simulink model "pato4CM00_23hz"  (R2015b)
settings: Solver=FixedStepDiscrete  StartTime=0.0  StopTime=1000  FixedStep=1/2048  RelTol=1e-3
settings Model: SimulationMode=external  ExtModeAutoUpdateStatusClock=off  Creator=root  LastModifiedBy=root
settings DataIOCC: LimitDataPoints=off  SaveFormat=Array  SignalLoggingSaveFormat=ModelDataLogs
settings OptimizationCC: ExpressionDepthLimit=2147483647  InitFltsAndDblsToZero=on
settings DebuggingCC: UnderspecifiedInitializationDetection=Classic  MergeDetectMultiDrivingBlocksExec=none  SolverPrmCheckMsg=warning  FcnCallInpInsideContextMsg=UseLocalSettings  StateNameClashWarn=warning
settings HardwareCC: ProdBitPerPointer=32  ProdLargestAtomicFloat=None  ProdIntDivRoundTo=Undefined  ProdEndianess=Unspecified  ProdWordSize=32  ProdHWDeviceType=32-bit Generic
settings RTWCC: SystemTargetFile=ectarget.tlc  MakeCommand="make_rtw OPTS=\"-DNETIF_ID=2\""  TemplateMakefile=ec_unix.tmf  Description=EtherCAT Real-Time Target for SOEM (IME Technologies 2008)
settings GRTTargetCC: GeneratePreprocessorConditionals=Disable all  CombineOutputUpdateFcns=off  GRTInterface=on  UseToolchainInfoCompliant=off  ExtMode=on
settings ConfigComp: CovModelRefEnable=Off  CovSFcnEnable=off

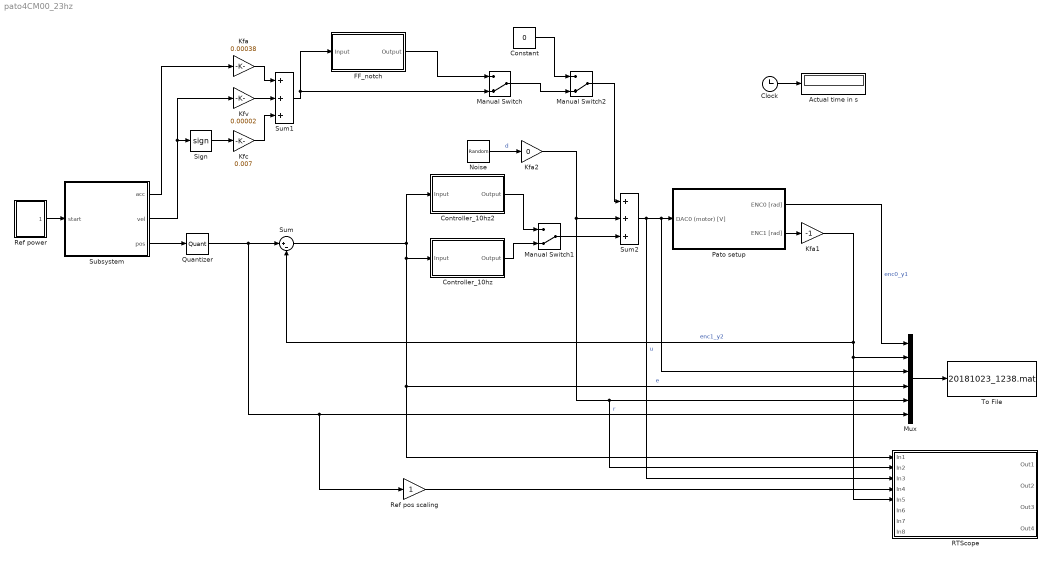
== system pato4CM00_23hz ==
  Actual time in s : Display
  Clock : Clock
  Constant : Constant  Value=0
  Controller_10hz : Subsystem  mask(Controller){Kp=100, Kv=0.005, notch_zeros=59, notch_damping_zeros=0.03, notch_poles=59, notch_damping_poles=0.5, roll_off_poles=200, roll_off_damping_poles=0.5}
      mask prompts: notch_zeros "Notch zeros [Hz]"; notch_damping_zeros "Notch damping zeros [-]"; notch_poles "Notch poles [Hz]"; notch_damping_poles "Notch damping poles [-]"; roll_off_poles "Roll-off poles [Hz]"; roll_off_damping_poles "Roll-off damping poles [-]"
      mask help:
      | The controller consists of three filters: a Kp/Kv, a notch and a roll-off filter.
      | You can edit the parameters below.
  Controller_10hz2 : Subsystem  mask(Controller){Kp=100, Kv=0.005, notch_zeros=59, notch_damping_zeros=0.03, notch_poles=59, notch_damping_poles=0.5, roll_off_poles=200, roll_off_damping_poles=0.5}
      mask prompts: notch_zeros "Notch zeros [Hz]"; notch_damping_zeros "Notch damping zeros [-]"; notch_poles "Notch poles [Hz]"; notch_damping_poles "Notch damping poles [-]"; roll_off_poles "Roll-off poles [Hz]"; roll_off_damping_poles "Roll-off damping poles [-]"
      mask help:
      | The controller consists of three filters: a Kp/Kv, a notch and a roll-off filter.
      | You can edit the parameters below.
  FF_notch : Subsystem  mask(Controller){Kp=100, Kv=0.005, notch_zeros=59, notch_damping_zeros=0.03, notch_poles=59, notch_damping_poles=0.5, roll_off_poles=200, roll_off_damping_poles=0.5}
      mask prompts: notch_zeros "Notch zeros [Hz]"; notch_damping_zeros "Notch damping zeros [-]"; notch_poles "Notch poles [Hz]"; notch_damping_poles "Notch damping poles [-]"; roll_off_poles "Roll-off poles [Hz]"; roll_off_damping_poles "Roll-off damping poles [-]"
      mask help:
      | The controller consists of three filters: a Kp/Kv, a notch and a roll-off filter.
      | You can edit the parameters below.
  Kfa : Gain  Gain=0.00038  SaturateOnIntegerOverflow=on  OutDataTypeStr=Inherit: Same as input  ParamDataTypeStr=Inherit: Same as input
  Kfa1 : Gain  Gain=-1  SaturateOnIntegerOverflow=on  OutDataTypeStr=Inherit: Same as input  ParamDataTypeStr=Inherit: Same as input
  Kfa2 : Gain  Gain=0  SaturateOnIntegerOverflow=on  OutDataTypeStr=Inherit: Same as input  ParamDataTypeStr=Inherit: Same as input
  Kfc : Gain  Gain=0.007  SaturateOnIntegerOverflow=on  OutDataTypeStr=Inherit: Same as input  ParamDataTypeStr=Inherit: Same as input
  Kfv : Gain  Gain=0.00002  SaturateOnIntegerOverflow=on  OutDataTypeStr=Inherit: Same as input  ParamDataTypeStr=Inherit: Same as input
  Manual Switch : ManualSwitch  CurrentSetting=0
  Manual Switch1 : ManualSwitch  CurrentSetting=0
  Manual Switch2 : ManualSwitch  CurrentSetting=0
  Mux : Mux  Inputs=6
  Noise : RandomNumber  Variance=0.1  SampleTime=0
  Pato setup : Subsystem  mask(Encoders){}
      mask help: Inc encoder positions 1-2 [rad] (see connector pannel).
  Quantizer : Quantizer  QuantizationInterval=(2*pi)/(500*4)
  RTScope : Subsystem  mask(RTScope){}
      settings: OpenFcn=rtscope
      mask Display: image(imread('rtscope2.jpg'))
  Ref pos scaling : Gain  SaturateOnIntegerOverflow=on  OutDataTypeStr=Inherit: Same as input  ParamDataTypeStr=Inherit: Same as input
  Ref power : Subsystem  mask(On/Off Switch){stat=On}
      mask prompts: stat "Switch"
      mask TypeOptions stat: On | Off
  Sign : Signum
  Subsystem : Subsystem  mask(Ref3){}
      settings: OpenFcn=global ref_part; cb_axes 1
      mask Display: disp('Ref3');
  Sum : Sum  Inputs=|+-  SaturateOnIntegerOverflow=on  InputSameDT=on  OutDataTypeStr=Inherit: Same as first input
  Sum1 : Sum  Description=sumff  Inputs=+++  SaturateOnIntegerOverflow=on  InputSameDT=on  OutDataTypeStr=Inherit: Same as first input
  Sum2 : Sum  Description=sumff  Inputs=+++  SaturateOnIntegerOverflow=on  InputSameDT=on  OutDataTypeStr=Inherit: Same as first input
  To File : ToFile  Filename=20181023_1238.mat
  wires:
  Subsystem/1(acc) -> Kfa/1
  Sum/1 -> Controller_10hz2/1(Input), Mux/4, RTScope/1(In1), Controller_10hz/1(Input)  "e"
  Sign/1 -> Kfc/1
  Ref power/1(On/Off) -> Subsystem/1(start)
  Ref pos scaling/1 -> RTScope/4(In4)
  Sum2/1 -> RTScope/3(In3), Mux/3, Pato setup/1(DAC0 (motor) [V])  "u"
  Subsystem/3(pos) -> Quantizer/1
  Subsystem/2(vel) -> Kfv/1, Sign/1
  Clock/1 -> Actual time in s/1
  Quantizer/1 -> Sum/1, Mux/6, Ref pos scaling/1  "r"
  Pato setup/2(ENC1 [rad]) -> Kfa1/1
  Kfa1/1 -> Sum/2, RTScope/5(In5), Mux/2  "enc1_y2"
  Mux/1 -> To File/1
  Pato setup/1(ENC0 [rad]) -> Mux/1  "enc0_y1"
  Kfa2/1 -> RTScope/2(In2), Mux/5, Sum2/2
  Noise/1 -> Kfa2/1  "d"
  Kfc/1 -> Sum1/3
  Kfv/1 -> Sum1/2
  Kfa/1 -> Sum1/1
  Sum1/1 -> FF_notch/1(Input), Manual Switch/2
  Manual Switch1/1 -> Sum2/3
  Manual Switch/1 -> Manual Switch2/2
  Manual Switch2/1 -> Sum2/1
  Constant/1 -> Manual Switch2/1
  Controller_10hz/1(Output) -> Manual Switch1/2
  Controller_10hz2/1(Output) -> Manual Switch1/1
  FF_notch/1(Output) -> Manual Switch/1

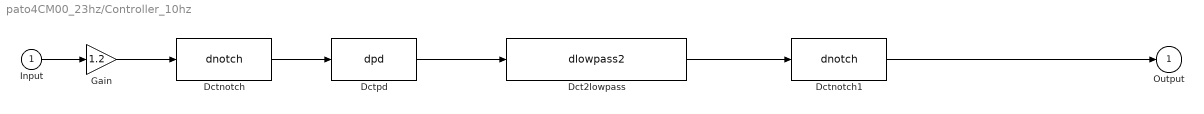
== system pato4CM00_23hz/Controller_10hz ==
  Input : Inport
  Dct2lowpass : S-Function  FunctionName=dlowpass2  Parameters=[f_den b_den 0.001]  SFunctionDeploymentMode=off  EnableBusSupport=off  mask(dctools){f_den=100, b_den=0.7}
      mask prompts: f_den "Pole [Hz]"; b_den "Damping pole [-]"
      mask help: This block implements a discrete time 2nd order lowpass filter.
      mask Display: disp('DCT 2nd order lowpass')
  Dctnotch : S-Function  FunctionName=dnotch  Parameters=[f_num b_num f_den b_den 0.001]  SFunctionDeploymentMode=off  EnableBusSupport=off  mask(dctools){f_num=58, b_num=0.005, f_den=59, b_den=0.5}
      mask prompts: f_num "Zero [Hz]"; b_num "Damping zero [-]"; f_den "Pole [Hz]"; b_den "Damping pole [-]"
      mask help: This block implements a dicrete time 2nd order notch filter.
      mask Display: disp('DCT notch')
  Dctnotch1 : S-Function  FunctionName=dnotch  Parameters=[f_num b_num f_den b_den 0.001]  SFunctionDeploymentMode=off  EnableBusSupport=off  mask(dctools){f_num=5, b_num=1, f_den=5, b_den=1}
      mask prompts: f_num "Zero [Hz]"; b_num "Damping zero [-]"; f_den "Pole [Hz]"; b_den "Damping pole [-]"
      mask help: This block implements a dicrete time 2nd order notch filter.
      mask Display: disp('DCT notch')
  Dctpd : S-Function  FunctionName=dpd  Parameters=[kp kv 0.001]  SFunctionDeploymentMode=off  EnableBusSupport=off  mask(dctools){kp=1, kv=0.03}
      mask help: This block implements a discrete time pd filter.
      mask Display: disp('DCT pd')
  Gain : Gain  Gain=1.2
  Output : Outport
  wires:
  Input/1 -> Gain/1
  Dct2lowpass/1 -> Dctnotch1/1
  Gain/1 -> Dctnotch/1
  Dctnotch/1 -> Dctpd/1
  Dctpd/1 -> Dct2lowpass/1
  Dctnotch1/1 -> Output/1

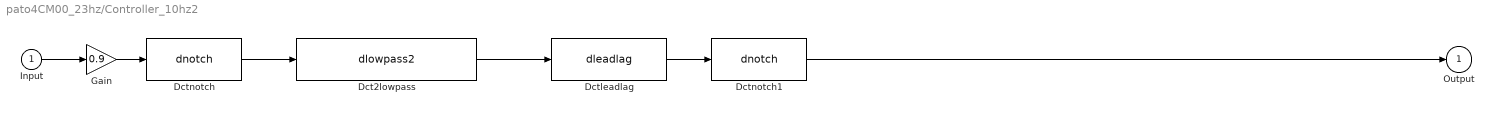
== system pato4CM00_23hz/Controller_10hz2 ==
  Input : Inport
  Dct2lowpass : S-Function  FunctionName=dlowpass2  Parameters=[f_den b_den 0.001]  SFunctionDeploymentMode=off  EnableBusSupport=off  mask(dctools){f_den=100, b_den=0.7}
      mask prompts: f_den "Pole [Hz]"; b_den "Damping pole [-]"
      mask help: This block implements a discrete time 2nd order lowpass filter.
      mask Display: disp('DCT 2nd order lowpass')
  Dctleadlag : S-Function  FunctionName=dleadlag  Parameters=[f_num f_den 0.001]  SFunctionDeploymentMode=off  EnableBusSupport=off  mask(dctools){f_num=11, f_den=30}
      mask prompts: f_num "Zero [Hz]"; f_den "Pole [Hz]"
      mask help: This block implements a discrete time leadlag filter.
      mask Display: disp('DCT leadlag')
  Dctnotch : S-Function  FunctionName=dnotch  Parameters=[f_num b_num f_den b_den 0.001]  SFunctionDeploymentMode=off  EnableBusSupport=off  mask(dctools){f_num=25.3, b_num=0.07, f_den=60, b_den=0.35}
      mask prompts: f_num "Zero [Hz]"; b_num "Damping zero [-]"; f_den "Pole [Hz]"; b_den "Damping pole [-]"
      mask help: This block implements a dicrete time 2nd order notch filter.
      mask Display: disp('DCT notch')
  Dctnotch1 : S-Function  FunctionName=dnotch  Parameters=[f_num b_num f_den b_den 0.001]  SFunctionDeploymentMode=off  EnableBusSupport=off  mask(dctools){f_num=5.5, b_num=0.6, f_den=7, b_den=1}
      mask prompts: f_num "Zero [Hz]"; b_num "Damping zero [-]"; f_den "Pole [Hz]"; b_den "Damping pole [-]"
      mask help: This block implements a dicrete time 2nd order notch filter.
      mask Display: disp('DCT notch')
  Gain : Gain  Gain=0.9
  Output : Outport
  wires:
  Input/1 -> Gain/1
  Gain/1 -> Dctnotch/1
  Dctnotch/1 -> Dct2lowpass/1
  Dctnotch1/1 -> Output/1
  Dct2lowpass/1 -> Dctleadlag/1
  Dctleadlag/1 -> Dctnotch1/1

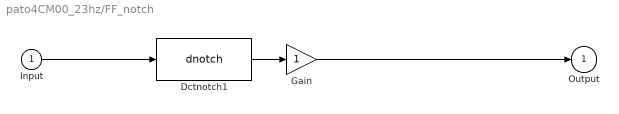
== system pato4CM00_23hz/FF_notch ==
  Input : Inport
  Dctnotch1 : S-Function  FunctionName=dnotch  Parameters=[f_num b_num f_den b_den 0.001]  SFunctionDeploymentMode=off  EnableBusSupport=off  mask(dctools){f_num=58, b_num=0.1, f_den=58, b_den=0.5}
      mask prompts: f_num "Zero [Hz]"; b_num "Damping zero [-]"; f_den "Pole [Hz]"; b_den "Damping pole [-]"
      mask help: This block implements a dicrete time 2nd order notch filter.
      mask Display: disp('DCT notch')
  Gain : Gain
  Output : Outport
  wires:
  Input/1 -> Dctnotch1/1
  Dctnotch1/1 -> Gain/1
  Gain/1 -> Output/1

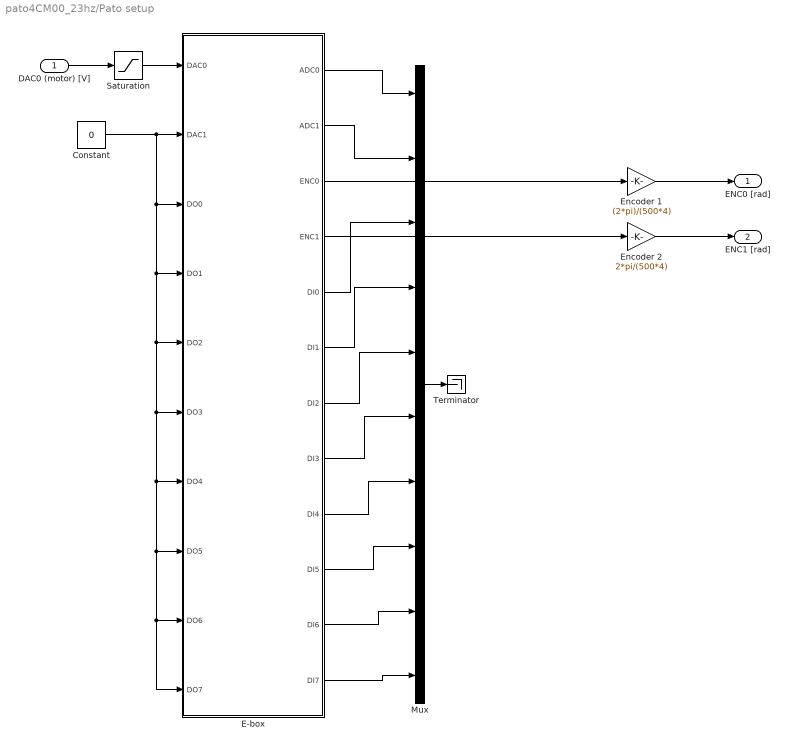
== system pato4CM00_23hz/Pato setup ==
  DAC0 (motor) [V] : Inport
  Constant : Constant  Value=0
  E-box : Subsystem  mask(E-box){link_id=0}
      mask prompts: link_id "Link id (>=0)"
  Encoder 1 : Gain  Gain=(2*pi)/(500*4)  SaturateOnIntegerOverflow=on  OutDataTypeStr=Inherit: Same as input  ParamDataTypeStr=Inherit: Same as input
  Encoder 2 : Gain  Gain=2*pi/(500*4)  SaturateOnIntegerOverflow=on  OutDataTypeStr=Inherit: Same as input  ParamDataTypeStr=Inherit: Same as input
  Mux : Mux  Inputs=10
  Saturation : Saturate  UpperLimit=2.5  LowerLimit=-2.5
  Terminator : Terminator
  ENC0 [rad] : Outport
  ENC1 [rad] : Outport  Port=2
  wires:
  E-box/3(ENC0) -> Encoder 1/1
  Encoder 1/1 -> ENC0 [rad]/1
  Encoder 2/1 -> ENC1 [rad]/1
  DAC0 (motor) [V]/1 -> Saturation/1
  Constant/1 -> E-box/2(DAC1), E-box/3(DO0), E-box/4(DO1), E-box/5(DO2), E-box/6(DO3), E-box/7(DO4), E-box/8(DO5), E-box/9(DO6), E-box/10(DO7)
  E-box/4(ENC1) -> Encoder 2/1
  E-box/1(ADC0) -> Mux/1
  E-box/2(ADC1) -> Mux/2
  E-box/5(DI0) -> Mux/3
  E-box/6(DI1) -> Mux/4
  E-box/7(DI2) -> Mux/5
  E-box/8(DI3) -> Mux/6
  E-box/9(DI4) -> Mux/7
  E-box/10(DI5) -> Mux/8
  E-box/11(DI6) -> Mux/9
  E-box/12(DI7) -> Mux/10
  Mux/1 -> Terminator/1
  Saturation/1 -> E-box/1(DAC0)

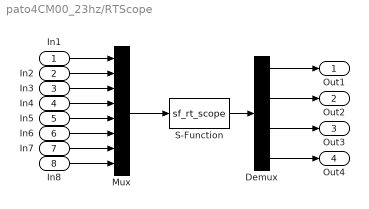
== system pato4CM00_23hz/RTScope ==
  In1 : Inport
  In2 : Inport  Port=2
  In3 : Inport  Port=3
  In4 : Inport  Port=4
  In5 : Inport  Port=5
  In6 : Inport  Port=6
  In7 : Inport  Port=7
  In8 : Inport  Port=8
  Demux : Demux
  Mux : Mux  Inputs=8
  S-Function : S-Function  FunctionName=sf_rt_scope  Parameters=4096  SFunctionDeploymentMode=off  EnableBusSupport=off
  Out1 : Outport
  Out2 : Outport  Port=2
  Out3 : Outport  Port=3
  Out4 : Outport  Port=4
  wires:
  In8/1 -> Mux/8
  In7/1 -> Mux/7
  In6/1 -> Mux/6
  In5/1 -> Mux/5
  In4/1 -> Mux/4
  In3/1 -> Mux/3
  In2/1 -> Mux/2
  In1/1 -> Mux/1
  Demux/4 -> Out4/1
  Demux/3 -> Out3/1
  Demux/2 -> Out2/1
  Demux/1 -> Out1/1
  S-Function/1 -> Demux/1
  Mux/1 -> S-Function/1

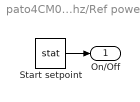
== system pato4CM00_23hz/Ref power ==
  Start setpoint : Constant  Value=stat
  On/Off : Outport
  wires:
  Start setpoint/1 -> On/Off/1

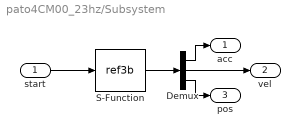
== system pato4CM00_23hz/Subsystem ==
  start : Inport
  Demux : Demux  Outputs=3
  S-Function : S-Function  FunctionName=ref3b  Parameters=ref_part  SFunctionDeploymentMode=off  EnableBusSupport=off
      settings: OpenFcn=global ref_part; r3g_main
  acc : Outport
  vel : Outport  Port=2
  pos : Outport  Port=3
  wires:
  S-Function/1 -> Demux/1
  Demux/1 -> acc/1
  Demux/2 -> vel/1
  Demux/3 -> pos/1
  start/1 -> S-Function/1

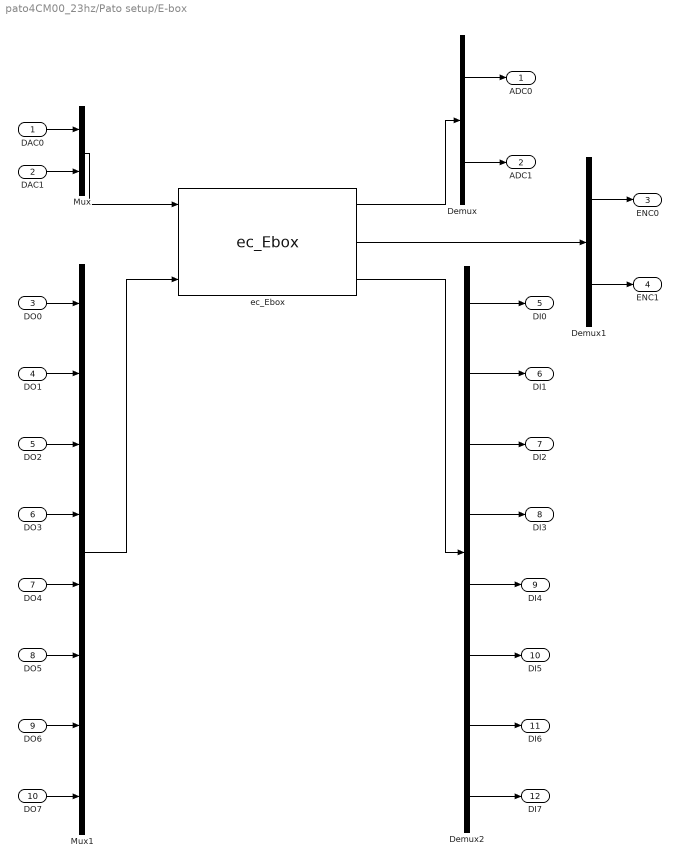
== system pato4CM00_23hz/Pato setup/E-box ==
  DAC0 : Inport
  DAC1 : Inport  Port=2
  DO0 : Inport  Port=3
  DO1 : Inport  Port=4
  DO2 : Inport  Port=5
  DO3 : Inport  Port=6
  DO4 : Inport  Port=7
  DO5 : Inport  Port=8
  DO6 : Inport  Port=9
  DO7 : Inport  Port=10
  Demux : Demux  Outputs=2
  Demux1 : Demux  Outputs=2
  Demux2 : Demux  Outputs=8
  Mux : Mux  Inputs=2
  Mux1 : Mux  Inputs=8
  ec_Ebox : S-Function  FunctionName=ec_Ebox  Parameters=link_id  SFunctionDeploymentMode=off  EnableBusSupport=off  mask{link_id=link_id}
      mask prompts: link_id "analog in id (start from 1)"
      mask Display:
      | port_label('output',1,'ADC')
      | port_label('output',2,'ENC')
      | port_label('output',3,'DI')
      | port_label('input',1,'DAC')
      | port_label('input',2,'PWM')
      | port_label('input',3,'DO')
  ADC0 : Outport
  ADC1 : Outport  Port=2
  ENC0 : Outport  Port=3
  ENC1 : Outport  Port=4
  DI0 : Outport  Port=5
  DI1 : Outport  Port=6
  DI2 : Outport  Port=7
  DI3 : Outport  Port=8
  DI4 : Outport  Port=9
  DI5 : Outport  Port=10
  DI6 : Outport  Port=11
  DI7 : Outport  Port=12
  wires:
  ec_Ebox/1 -> Demux/1
  Demux/1 -> ADC0/1
  Demux/2 -> ADC1/1
  Demux1/1 -> ENC0/1
  Demux1/2 -> ENC1/1
  ec_Ebox/2 -> Demux1/1
  Mux/1 -> ec_Ebox/1
  DAC0/1 -> Mux/1
  DAC1/1 -> Mux/2
  ec_Ebox/3 -> Demux2/1
  Demux2/1 -> DI0/1
  Demux2/2 -> DI1/1
  Demux2/3 -> DI2/1
  Demux2/4 -> DI3/1
  Demux2/5 -> DI4/1
  Demux2/6 -> DI5/1
  Demux2/7 -> DI6/1
  Demux2/8 -> DI7/1
  Mux1/1 -> ec_Ebox/3
  DO0/1 -> Mux1/1
  DO1/1 -> Mux1/2
  DO2/1 -> Mux1/3
  DO3/1 -> Mux1/4
  DO4/1 -> Mux1/5
  DO5/1 -> Mux1/6
  DO6/1 -> Mux1/7
  DO7/1 -> Mux1/8
